simulink model "Host"  (R2024b)
settings: Solver=ode14x  StartTime=0.0  StopTime=inf  FixedStep=hostParams.Ts  RelTol=1e-3
PreLoadFcn:
  | % Load scenario parameters if not already loaded
  | if ~exist('hostParams', 'var')
  |     hostParams = helperScenarioParams;
  | end
  | 
  | % Load vehicle parameters if not already loaded
  | if ~exist('vehicleParams', 'var')
  |     vehicleParams = helperVehicleParams;
  | end
  | 
  | % Load PathFollower parameters if not already loaded
  | if ~exist('controllerParams', 'var')
  |     controllerParams = helperPathFollowerParams;
  | end
  | 
  | % Set IP addresses to local computer if they are not provided
  | if ~exist('ipAddress', 'var')
  |     ipAddress = helperIPAddresses;
  | end
StopFcn:
  | close(gcf)
  | clear functions
libraries: simulink x5, slrealtimeutilitieslib x3, slrealtimeiplib x3, offroadsim3dlib x1, sim3dlib x1, sim3dautolib x1
settings Model: Creator=smaddina  LastModifiedBy=demo-user2
settings SolverCC: PositivePriorityOrder=on
settings OptimizationCC: BlockReduction=off  DefaultParameterBehavior=Inlined  EnhancedBackFolding=on  PassReuseOutputArgsAs=Individual arguments  ZeroExternalMemoryAtStartup=off  ZeroInternalMemoryAtStartup=off  MaxStackSize=64  OptimizeBlockOrder=speed  DifferentSizesBufferReuse=on  OptimizationCustomize=off  EfficientTunableParamExpr=on
settings DebuggingCC: TasksWithSamePriorityMsg=none  ParameterTunabilityLossMsg=error
settings SFSimCC: MATLABDynamicMemAlloc=off
settings RTWCC: Description=Embedded Coder  SystemTargetFile=ert.tlc  TemplateMakefile=ert_default_tmf  Toolchain=Colcon Tools  BuildConfiguration=Faster Runs  CodeExecutionProfiling=on
settings CodeAppCC: ForceParamTrailComments=on  IgnoreCustomStorageClasses=off  MaxIdLength=95  OperatorAnnotations=on  SimulinkDataObjDesc=on  SFDataObjDesc=on  InsertBlockDesc=on
settings ERTTargetCC: RootIOFormat=Structure reference  ERTCustomFileTemplate=example_file_process.tlc

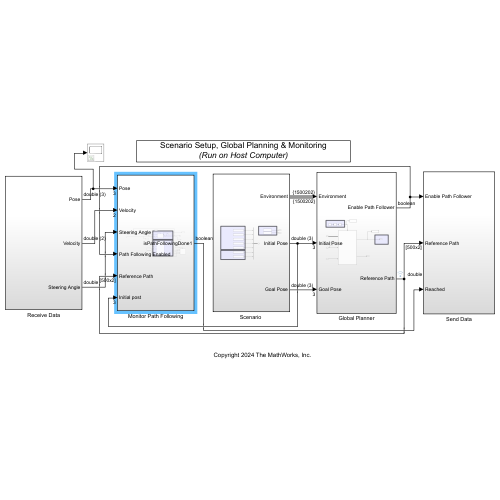
[thumbnail: Simulink's stored preview of the top-level diagram]
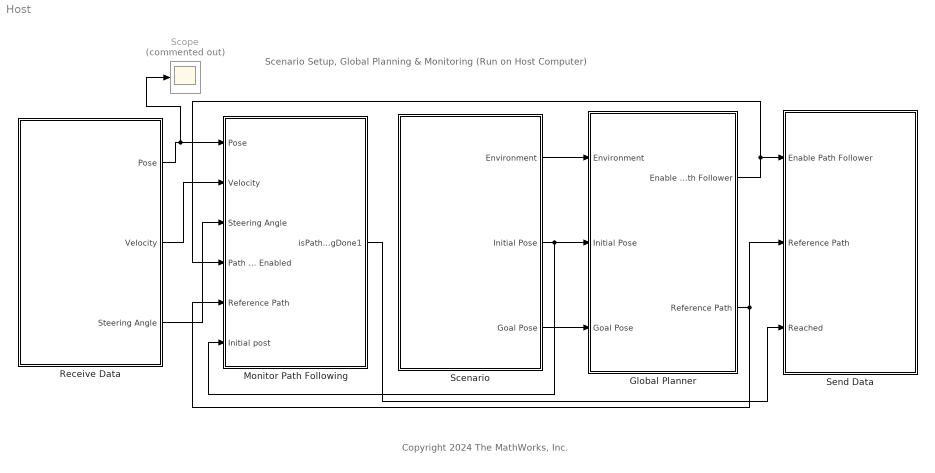
== system Host ==
  note: Copyright 2024 The MathWorks, Inc.
  note: Scenario Setup, Global Planning & Monitoring
      | (Run on Host Computer)
  Global Planner : Subsystem
  Monitor Path Following : Subsystem
  Receive Data : Subsystem
  "Scenario " : Subsystem
  Scope : Scope  Commented=on
  Send Data : Subsystem
  wires:
  Global Planner/2(Reference Path) -> Send Data/2(Reference Path), Monitor Path Following/5(Reference Path)
  Global Planner/1(Enable Path Follower) -> Send Data/1(Enable Path Follower), Monitor Path Following/4(Path Following Enabled)
  "Scenario "/1(Environment) -> Global Planner/1(Environment)
  "Scenario "/2(Initial Pose) -> Monitor Path Following/6(Initial post), Global Planner/2(Initial Pose)
  "Scenario "/3(Goal Pose) -> Global Planner/3(Goal Pose)
  Receive Data/1(Pose) -> Scope/1, Monitor Path Following/1(Pose)
  Receive Data/2(Velocity) -> Monitor Path Following/2(Velocity)
  Receive Data/3(Steering Angle) -> Monitor Path Following/3(Steering Angle)
  Monitor Path Following/1(isPathFollowingDone1) -> Send Data/3(Reached)

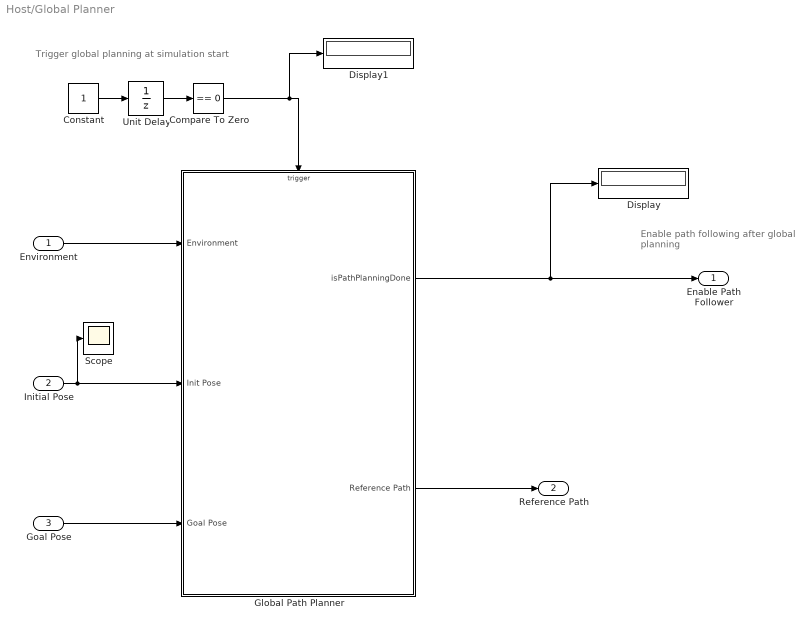
== system Host/Global Planner ==
  note: Enable path following
      | after global planning
  note: Trigger global planning at simulation start
  Environment : Inport
  Initial Pose : Inport  Port=2
  Goal Pose : Inport  Port=3
  Compare To Zero : simulink/Logic and Bit Operations/Compare To Zero  relop===  OutDataTypeStr=boolean
  Constant : Constant
  Display : Display
  Display1 : Display
  Global Path Planner : Subsystem  TreatAsAtomicUnit=on
  Scope : Scope
  Unit Delay : UnitDelay  SampleTime=-1  HasFrameUpgradeWarning=on
  Enable Path Follower : Outport
  Reference Path : Outport  Port=2
  wires:
  Unit Delay/1 -> Compare To Zero/1
  Global Path Planner/2(Reference Path) -> Reference Path/1
  Compare To Zero/1 -> Display1/1, Global Path Planner/Trigger
  Constant/1 -> Unit Delay/1
  Global Path Planner/1(isPathPlanningDone) -> Display/1, Enable Path Follower/1
  Environment/1 -> Global Path Planner/1(Environment)
  Initial Pose/1 -> Scope/1, Global Path Planner/2(Init Pose)
  Goal Pose/1 -> Global Path Planner/3(Goal Pose)

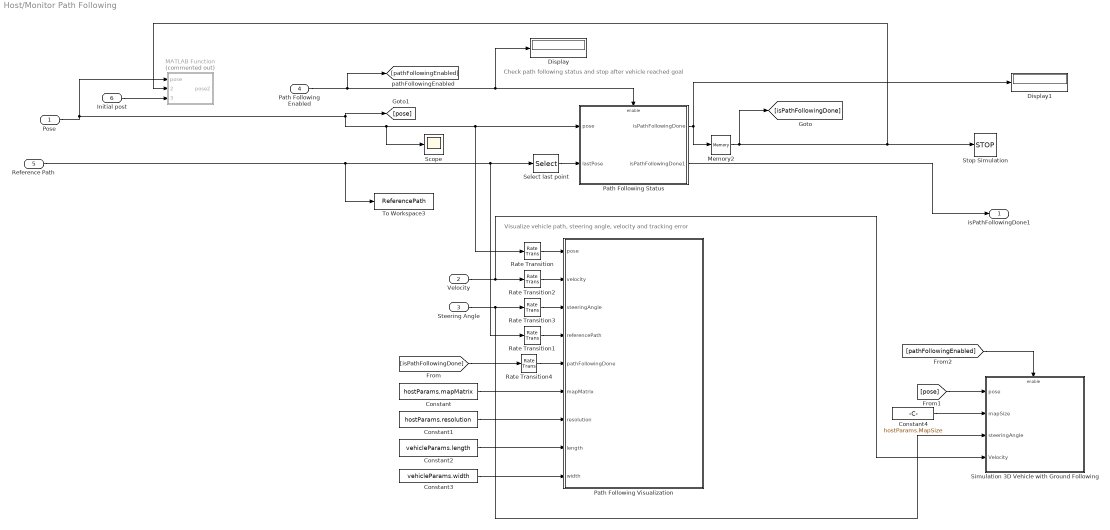
== system Host/Monitor Path Following ==
  note: Visualize vehicle path, steering angle, velocity and tracking error
  note: Check path following status and stop after vehicle reached goal
  Pose : Inport
  Velocity : Inport  Port=2
  Steering Angle : Inport  Port=3
  Path Following Enabled : Inport  Port=4
  Reference Path : Inport  Port=5
  Initial post : Inport  Port=6
  Constant : Constant  Value=hostParams.mapMatrix
  Constant1 : Constant  Value=hostParams.resolution
  Constant2 : Constant  Value=vehicleParams.length
  Constant3 : Constant  Value=vehicleParams.width
  Constant4 : Constant  Value=hostParams.MapSize
  Display : Display
  Display1 : Display
  MATLAB Function : MATLAB Function  Commented=on  TreatAsAtomicUnit=on
  Memory2 : Memory  InitialCondition=false
  Path Following Status : Subsystem
  Path Following Visualization : MATLAB Function  TreatAsAtomicUnit=on  SystemSampleTime=0.2
  Rate Transition : RateTransition  InitialCondition=hostParams.initPose
  Rate Transition1 : RateTransition
  Rate Transition2 : RateTransition
  Rate Transition3 : RateTransition
  Rate Transition4 : RateTransition  InitialCondition=false
  Scope : Scope
  Select last point : Selector  NumberOfDimensions=2  InputPortWidth=3  IndexOptions=Index vector (dialog),Index vector (dialog)  Indices=hostParams.referencePathSize,[1:2]  OutputSizes=1,1
  Simulation 3D Vehicle with Ground Following : Subsystem
  Stop Simulation : Stop
  To Workspace3 : ToWorkspace  VariableName=ReferencePath  SaveFormat=Timeseries  SampleTime=-1
      settings: MaxDataPoints=1
  isPathFollowingDone1 : Outport
  wires:
  Select last point/1 -> Path Following Status/2(lastPose)
  Path Following Status/1(isPathFollowingDone) -> Memory2/1, Display1/1
  Path Following Enabled/1 -> [pathFollowingEnabled], Display/1, Path Following Status/Enable
  Rate Transition/1 -> Path Following Visualization/1(pose)
  Rate Transition1/1 -> Path Following Visualization/4(referencePath)
  Velocity/1 -> Simulation 3D Vehicle with Ground Following/4(Velocity), Rate Transition2/1
  Steering Angle/1 -> Simulation 3D Vehicle with Ground Following/3(steeringAngle), Rate Transition3/1
  Rate Transition2/1 -> Path Following Visualization/2(velocity)
  Rate Transition3/1 -> Path Following Visualization/3(steeringAngle)
  [isPathFollowingDone] -> Rate Transition4/1
  Rate Transition4/1 -> Path Following Visualization/5(pathFollowingDone)
  Constant/1 -> Path Following Visualization/6(mapMatrix)
  Constant1/1 -> Path Following Visualization/7(resolution)
  Constant2/1 -> Path Following Visualization/8(length)
  Constant3/1 -> Path Following Visualization/9(width)
  [pose] -> Simulation 3D Vehicle with Ground Following/1(pose)
  Constant4/1 -> Simulation 3D Vehicle with Ground Following/2(mapSize)
  [pathFollowingEnabled] -> Simulation 3D Vehicle with Ground Following/Enable
  Reference Path/1 -> Select last point/1, Rate Transition1/1, To Workspace3/1
  Pose/1 -> Scope/1, Path Following Status/1(pose), Rate Transition/1, [pose], MATLAB Function/1(pose)
  Initial post/1 -> MATLAB Function/3(initpose)
  Memory2/1 -> Stop Simulation/1, MATLAB Function/2(endoftraj), [isPathFollowingDone]
  Path Following Status/2(isPathFollowingDone1) -> isPathFollowingDone1/1

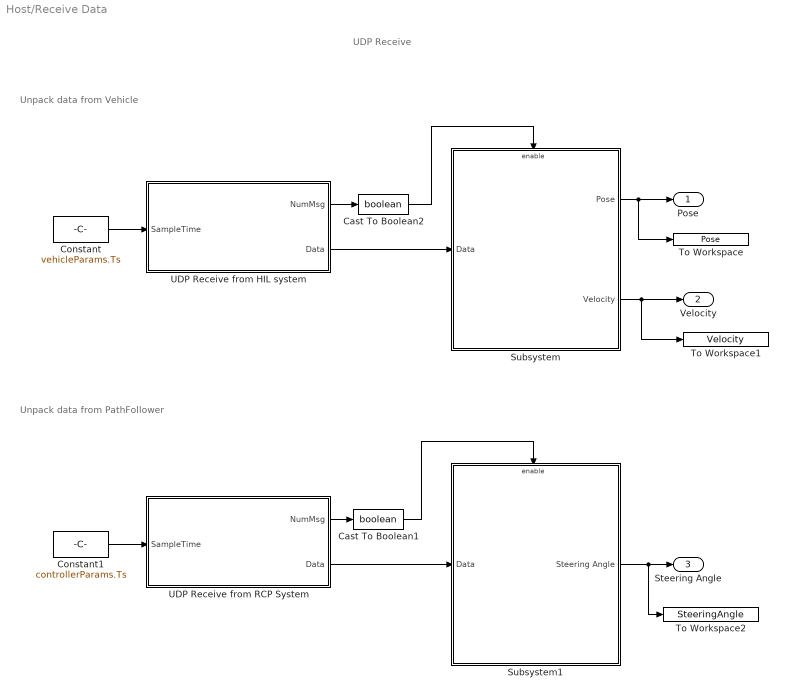
== system Host/Receive Data ==
  note: Unpack data from PathFollower
  note: Unpack data from Vehicle
  note: UDP Receive
  Cast To Boolean1 : DataTypeConversion  OutDataTypeStr=boolean  SaturateOnIntegerOverflow=off  RndMeth=Floor
  Cast To Boolean2 : DataTypeConversion  OutDataTypeStr=boolean  SaturateOnIntegerOverflow=off  RndMeth=Floor
  Constant : Constant  Value=vehicleParams.Ts  SampleTime=vehicleParams.Ts
  Constant1 : Constant  Value=controllerParams.Ts  SampleTime=controllerParams.Ts
  Subsystem : Subsystem
  Subsystem1 : Subsystem
  To Workspace : ToWorkspace  VariableName=Pose  SaveFormat=Timeseries  SampleTime=0.01
  To Workspace1 : ToWorkspace  VariableName=Velocity  SaveFormat=Timeseries  SampleTime=0.01
  To Workspace2 : ToWorkspace  VariableName=SteeringAngle  SaveFormat=Timeseries  SampleTime=0.01
  UDP Receive from HIL system : Subsystem  TreatAsAtomicUnit=on
  UDP Receive from RCP System : Subsystem  TreatAsAtomicUnit=on
  Pose : Outport
  Velocity : Outport  Port=2
  Steering Angle : Outport  Port=3
  wires:
  UDP Receive from HIL system/1(NumMsg) -> Cast To Boolean2/1
  UDP Receive from HIL system/2(Data) -> Subsystem/1(Data)
  Subsystem/1(Pose) -> Pose/1, To Workspace/1
  Subsystem/2(Velocity) -> Velocity/1, To Workspace1/1
  Cast To Boolean2/1 -> Subsystem/Enable
  Subsystem1/1(Steering Angle) -> Steering Angle/1, To Workspace2/1
  Constant/1 -> UDP Receive from HIL system/1(SampleTime)
  UDP Receive from RCP System/2(Data) -> Subsystem1/1(Data)
  Constant1/1 -> UDP Receive from RCP System/1(SampleTime)
  UDP Receive from RCP System/1(NumMsg) -> Cast To Boolean1/1
  Cast To Boolean1/1 -> Subsystem1/Enable

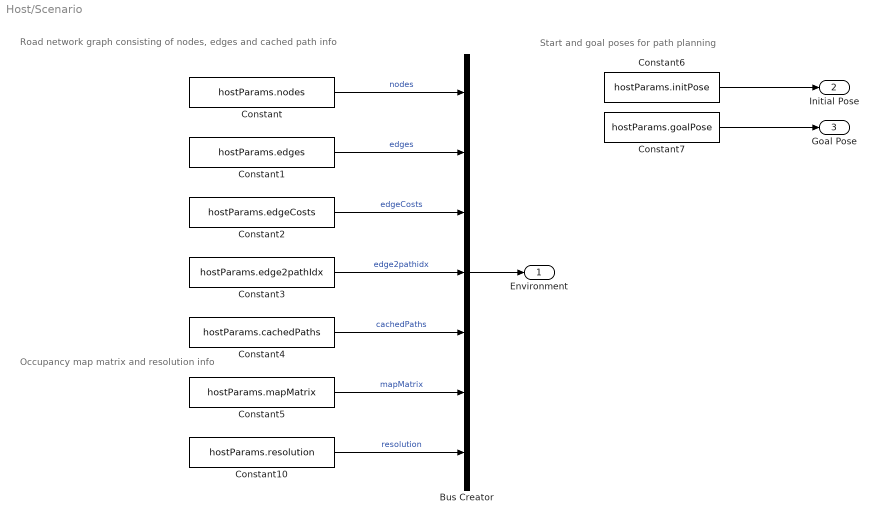
== system Host/Scenario  ==
  note: Start and goal poses for path planning
  note: Occupancy map matrix and
      | resolution info
  note: Road network graph consisting
      | of nodes, edges and cached path info
  Bus Creator : BusCreator  Inputs=7
  Constant : Constant  Value=hostParams.nodes
  Constant1 : Constant  Value=hostParams.edges
  Constant10 : Constant  Value=hostParams.resolution
  Constant2 : Constant  Value=hostParams.edgeCosts
  Constant3 : Constant  Value=hostParams.edge2pathIdx
  Constant4 : Constant  Value=hostParams.cachedPaths
  Constant5 : Constant  Value=hostParams.mapMatrix
  Constant6 : Constant  Value=hostParams.initPose
  Constant7 : Constant  Value=hostParams.goalPose
  Environment : Outport
  Initial Pose : Outport  Port=2
  Goal Pose : Outport  Port=3
  wires:
  Constant/1 -> Bus Creator/1  "nodes"
  Constant1/1 -> Bus Creator/2  "edges"
  Constant2/1 -> Bus Creator/3  "edgeCosts"
  Constant4/1 -> Bus Creator/5  "cachedPaths"
  Constant3/1 -> Bus Creator/4  "edge2pathidx"
  Constant5/1 -> Bus Creator/6  "mapMatrix"
  Constant10/1 -> Bus Creator/7  "resolution"
  Bus Creator/1 -> Environment/1
  Constant7/1 -> Goal Pose/1
  Constant6/1 -> Initial Pose/1

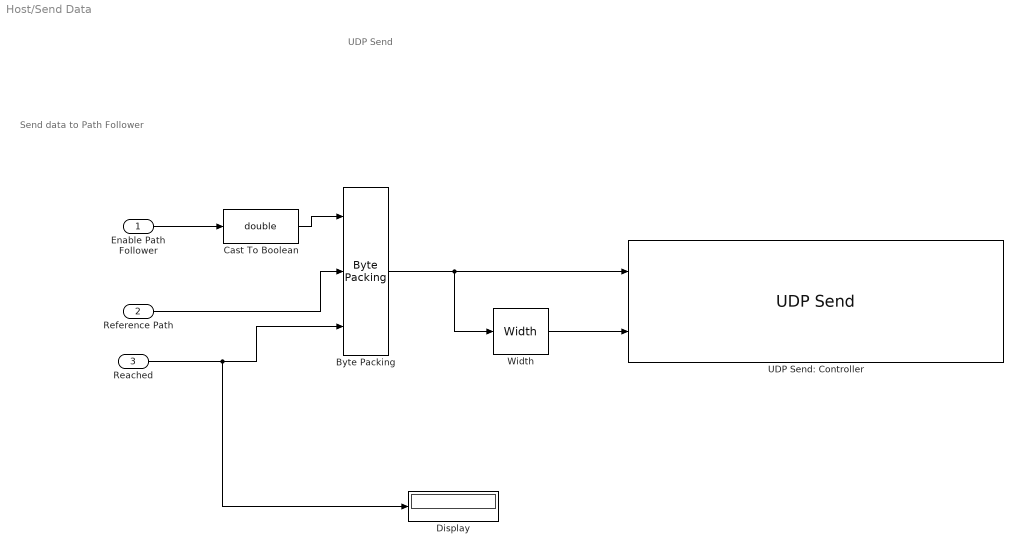
== system Host/Send Data ==
  note: Send data to Path Follower
  note: UDP Send
  Enable Path Follower : Inport
  Reference Path : Inport  Port=2
  Reached : Inport  Port=3
  Byte Packing : slrealtimeutilitieslib/Byte Packing  MaskPackedDataType=uint8  MaskUnpackedDataTypes="{'double',  'double','boolean'}"  MaskAlignment=1
  Cast To Boolean : DataTypeConversion  OutDataTypeStr=double  SaturateOnIntegerOverflow=off  RndMeth=Floor
  Display : Display
  UDP Send: Controller : slrealtimeiplib/UDP Send  useHostTargetConn=on  toAddress=ipAddress.rcpSystem  toPort=8001  sampleTime=-1  enableMessage=off  localPort=-1
  Width : Width
  wires:
  Width/1 -> UDP Send: Controller/2
  Byte Packing/1 -> UDP Send: Controller/1, Width/1
  Reference Path/1 -> Byte Packing/2
  Enable Path Follower/1 -> Cast To Boolean/1
  Cast To Boolean/1 -> Byte Packing/1
  Reached/1 -> Display/1, Byte Packing/3

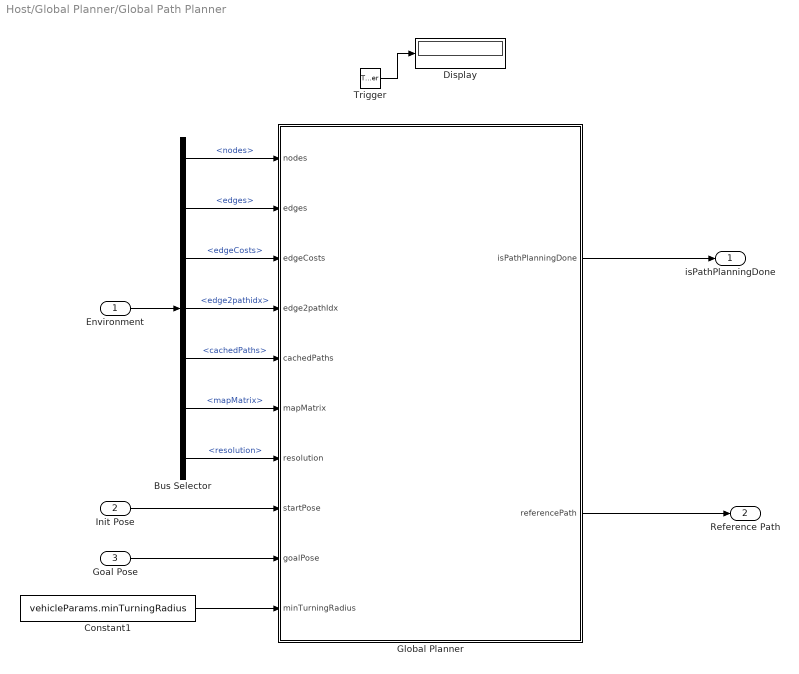
== system Host/Global Planner/Global Path Planner ==
  Environment : Inport
  Init Pose : Inport  Port=2
  Goal Pose : Inport  Port=3
  Trigger : TriggerPort  TriggerType=falling  VariantControl=(inherit)  ShowOutputPort=on  PortDimensions=1
  Bus Selector : BusSelector  OutputSignals=nodes,edges,edgeCosts,edge2pathidx,cachedPaths,mapMatrix,resolution
  Constant1 : Constant  Value=vehicleParams.minTurningRadius
  Display : Display
  Global Planner : MATLAB Function  InitFcn=referencePathSize = hostParams.referencePathSize;  TreatAsAtomicUnit=on
  isPathPlanningDone : Outport
  Reference Path : Outport  Port=2
  wires:
  Global Planner/1(isPathPlanningDone) -> isPathPlanningDone/1
  Global Planner/2(referencePath) -> Reference Path/1
  Environment/1 -> Bus Selector/1
  Bus Selector/2 -> Global Planner/2(edges)  "<edges>"
  Bus Selector/1 -> Global Planner/1(nodes)  "<nodes>"
  Bus Selector/3 -> Global Planner/3(edgeCosts)  "<edgeCosts>"
  Bus Selector/4 -> Global Planner/4(edge2pathIdx)  "<edge2pathidx>"
  Bus Selector/5 -> Global Planner/5(cachedPaths)  "<cachedPaths>"
  Bus Selector/6 -> Global Planner/6(mapMatrix)  "<mapMatrix>"
  Bus Selector/7 -> Global Planner/7(resolution)  "<resolution>"
  Init Pose/1 -> Global Planner/8(startPose)
  Goal Pose/1 -> Global Planner/9(goalPose)
  Constant1/1 -> Global Planner/10(minTurningRadius)
  Trigger/1 -> Display/1

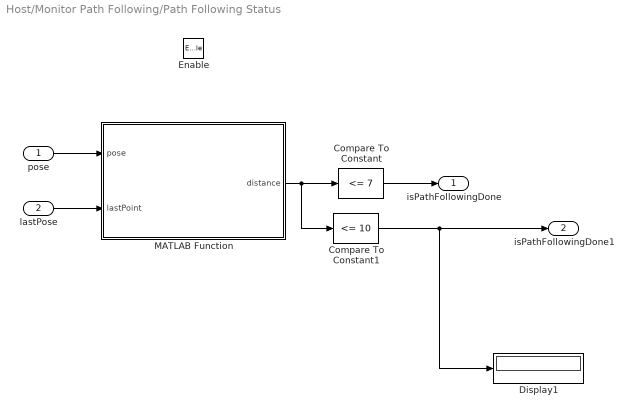
== system Host/Monitor Path Following/Path Following Status ==
  pose : Inport
  lastPose : Inport  Port=2
  Enable : EnablePort
  Compare To Constant : simulink/Logic and Bit Operations/Compare To Constant  relop=<=  const=7  OutDataTypeStr=boolean
  Compare To Constant1 : simulink/Logic and Bit Operations/Compare To Constant  relop=<=  const=10  OutDataTypeStr=boolean
  Display1 : Display
  MATLAB Function : MATLAB Function  TreatAsAtomicUnit=on
  isPathFollowingDone : Outport
  isPathFollowingDone1 : Outport  Port=2
  wires:
  lastPose/1 -> MATLAB Function/2(lastPoint)
  pose/1 -> MATLAB Function/1(pose)
  Compare To Constant/1 -> isPathFollowingDone/1
  MATLAB Function/1(distance) -> Compare To Constant1/1, Compare To Constant/1
  Compare To Constant1/1 -> Display1/1, isPathFollowingDone1/1

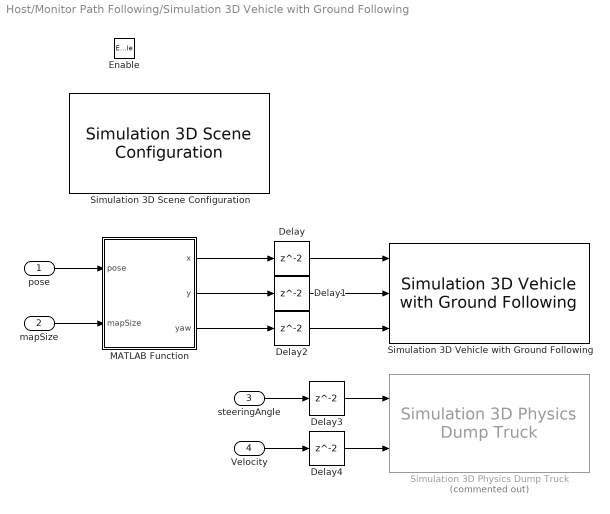
== system Host/Monitor Path Following/Simulation 3D Vehicle with Ground Following ==
  pose : Inport
  mapSize : Inport  Port=2
  steeringAngle : Inport  Port=3
  Velocity : Inport  Port=4
  Enable : EnablePort
  Delay{,1..4} (5 alike) : Delay
  MATLAB Function : MATLAB Function  TreatAsAtomicUnit=on
  Simulation 3D Physics Dump Truck : offroadsim3dlib/Simulation 3D Physics Dump Truck  Commented=on  TruckType=Standard Dump Truck  TruckColor=Yellow  ActorName=SimulinkVehicle2  InitTruckTrans=[0 0 0]  InitTruckRot=[0 0 0]  InitTruckVel=0  InitTruckAccel=0  InitTruckBedAng=0  EnbAccelInp=off  EnbFootBrakInp=off  EnbLifAngInp=off  EnbTruckTransOut=off  EnbTruckRotOut=off  EnbTruckVelOut=off  EnbTruckAngVelOut=off  EnbTruckBedTransOut=off  EnbTruckBedRotOut=off  EnbTruckBedAngOut=off  SampleTime=0.01  ActorType=SimulinkVehicle  ID=2  aMode=6  ActorTag=SimulinkVehicle2  Mesh=DumpTruck
  Simulation 3D Scene Configuration : sim3dlib/Simulation 3D Scene Configuration  Priority=0  ProjectFormat=Default Scenes  SceneDesc=Offroad pit mining scene  ProjectName=C:\Program Files\MATLAB\R2024b\toolbox\shared\sim3d_projects\automotive_project_windows\UE\WindowsNoEditor\VehicleSimulation.exe  ScenePath=/Game/Maps/HwStrght  EnableOpenDRIVE=off  vehTagList={'Custom';'Scene Origin';'SimulinkVehicle1'}  vehTag=SimulinkVehicle1  FreeCameraInitialTranslation=[0, 0, 0]  FreeCameraDefaultInitialTranslation=[-6, 0, 2]  FreeCameraInitialRotation=[0, 0, 0]  FreeCameraDefaultInitialRotation=[0, -15, 0]  OpVisEn=off  Ts=0.02  EnableWindow=on  EnableRemoteAccess=off  EnableWeather=off  SunAzimuth=90  SunAltitude=40.0  EnableGeospatialSun=off  Latitude=0  Longitude=0  Date=2023-01-01  Time=10:30:00  GeoTimeZone=-5.0  SunDaylightSaving=off  wind=1  clouds=10  EnableVolumetricClouds=off  CloudCoverage=0  CloudAltitude=6  fog=0  rain=0  RaindropsEffect=off  SnowDensity=0  EnableGeospatial=off  UseTrueOrigin=off  OriginHeight=200  OriginLatitude=40.744652  OriginLongitude=-73.988864  MapStyle=Aerial  AdditionalAssetIDs=[]  UseAdvancedSunSky=off  SolarTime=11  TimeZone=-5  Day=21  Month=9  Year=2022  UseDaylightSavingTime=on  DSTStartDay=10  DSTStartMonth=3  DSTEndDay=3  DSTEndMonth=11  DSTSwitchHour=2  sensorTag=MainCamera1  sensorId=1  sensorName=MainCamera1  mountLoc=Origin  offsetFlag=off  tmountOffset=[0, 0, 0]  rmountOffset=[0, 0, 0]  HorizontalResolution=1280  VerticalResolution=720  HorizontalFOV=60  mountPoint=[0 0 0]  mountOrientation=[0 0 0]  aMode=6  ID=1  GeoTrigger=Inactive
      settings: LibrarySourceBlock=offroadsim3dlib/Simulation 3D Scene Configuration
  Simulation 3D Vehicle with Ground Following : sim3dautolib/Simulation 3D Vehicle with Ground Following  Priority=1  PassVehMesh=Small pickup truck  MeshPath=/MathWorksAutomotiveContent/Vehicles/Muscle/Meshes/SK_MuscleCar.SK_MuscleCar  TrackWidth=1.9  WheelBase=3  WheelRadius=0.35  VehColor=Red  InitialPos=hostParams.Sim3DInitTranslation  InitialRot=hostParams.Sim3DInitRotation  ActorName=SimulinkVehicle1  SampleTime=hostParams.Ts  ActorType=SimulinkVehicle  ID=1  aMode=5  ActorTag=SimulinkVehicle1  CoordinateScheme=ISO  VehLightsControl=off  HeadlightColor=[ 1, 1, 1 ]  HighBeamIntensity=100000  LowBeamIntensity=60000  HighBeamConeAngle=70  LowBeamConeAngle=70  LeftHeadlightOrientation=[ 0, 0 ]  RightHeadlightOrientation=[ 0, 0 ]  BrakelightIntensity=500  ReverselightIntensity=500  SignallightIntensity=500  SignallightPeriod=1  SignalPulseWidth=50  TransformOutportEnabled=off
      settings: LibrarySourceBlock=sl3dlib/Simulation 3D/Actors/Simulation 3D Vehicle with Ground Following
  wires:
  mapSize/1 -> MATLAB Function/2(mapSize)
  pose/1 -> MATLAB Function/1(pose)
  MATLAB Function/1(x) -> Delay/1
  MATLAB Function/2(y) -> Delay1/1
  MATLAB Function/3(yaw) -> Delay2/1
  Delay/1 -> Simulation 3D Vehicle with Ground Following/1
  Delay1/1 -> Simulation 3D Vehicle with Ground Following/2
  Delay2/1 -> Simulation 3D Vehicle with Ground Following/3
  steeringAngle/1 -> Delay3/1
  Velocity/1 -> Delay4/1
  Delay3/1 -> Simulation 3D Physics Dump Truck/1
  Delay4/1 -> Simulation 3D Physics Dump Truck/2

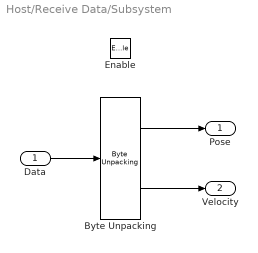
== system Host/Receive Data/Subsystem ==
  Data : Inport
  Enable : EnablePort
  Byte Unpacking : slrealtimeutilitieslib/Byte Unpacking  MaskUnpackedDataTypes={ 'double', 'double'}  MaskUnpackedDataSizes={3, 2}  MaskAlignment=1
  Pose : Outport
  Velocity : Outport  Port=2
  wires:
  Byte Unpacking/2 -> Velocity/1
  Data/1 -> Byte Unpacking/1
  Byte Unpacking/1 -> Pose/1

== system Host/Receive Data/Subsystem1 ==
  Data : Inport
  Enable : EnablePort
  Acceleration : Terminator
  Byte Unpacking : slrealtimeutilitieslib/Byte Unpacking  MaskUnpackedDataTypes="{'double',  'double'}"  MaskUnpackedDataSizes={1, 1}  MaskAlignment=1
  Steering Angle : Outport
  wires:
  Data/1 -> Byte Unpacking/1
  Byte Unpacking/2 -> Steering Angle/1
  Byte Unpacking/1 -> Acceleration/1

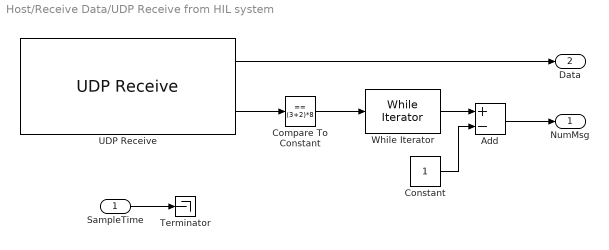
== system Host/Receive Data/UDP Receive from HIL system ==
  SampleTime : Inport
  Add : Sum  Inputs=+-
  Compare To Constant : simulink/Logic and Bit Operations/Compare To Constant  relop===  const=(3+2)*8  OutDataTypeStr=boolean
  Constant : Constant
  Terminator : Terminator
  UDP Receive : slrealtimeiplib/UDP Receive  useHostTargetConn=on  ipAddress=10.10.10.15  localPort=8005  rcvWidth=(3+2)*8  rcvFmAny=on  fmAddress='10.10.10.10'  sampleTime=-1  enableMessage=off  maxPackets=1
  While Iterator : WhileIterator  WhileBlockType=do-while  ShowIterationPort=on
  NumMsg : Outport
  Data : Outport  Port=2
  wires:
  Compare To Constant/1 -> While Iterator/1
  UDP Receive/1 -> Data/1
  UDP Receive/2 -> Compare To Constant/1
  Add/1 -> NumMsg/1
  While Iterator/1 -> Add/1
  Constant/1 -> Add/2
  SampleTime/1 -> Terminator/1

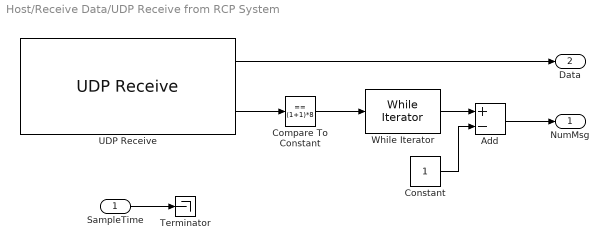
== system Host/Receive Data/UDP Receive from RCP System ==
  SampleTime : Inport
  Add : Sum  Inputs=+-
  Compare To Constant : simulink/Logic and Bit Operations/Compare To Constant  relop===  const=(1+1)*8  OutDataTypeStr=boolean
  Constant : Constant
  Terminator : Terminator
  UDP Receive : slrealtimeiplib/UDP Receive  useHostTargetConn=on  ipAddress=10.10.10.15  localPort=8004  rcvWidth=(1+1)*8  rcvFmAny=on  fmAddress='10.10.10.10'  sampleTime=-1  enableMessage=off  maxPackets=1
  While Iterator : WhileIterator  WhileBlockType=do-while  ShowIterationPort=on
  NumMsg : Outport
  Data : Outport  Port=2
  wires:
  Compare To Constant/1 -> While Iterator/1
  UDP Receive/1 -> Data/1
  UDP Receive/2 -> Compare To Constant/1
  Add/1 -> NumMsg/1
  While Iterator/1 -> Add/1
  Constant/1 -> Add/2
  SampleTime/1 -> Terminator/1

== matlab function Host/Global Planner/Global Path Planner/Global Planner ==
  data: isPathPlanningDone output; nodes input; edges input; edgeCosts input; edge2pathIdx input; cachedPaths input; mapMatrix input; resolution input; startPose input; goalPose input; referencePath output size=[hostParams.referencePathSize,2]; minTurningRadius input; referencePathSize parameter
function [isPathPlanningDone, referencePath] = planRoadNetworkPath(...
    nodes, edges, edgeCosts, edge2pathIdx, cachedPaths,...
    mapMatrix, resolution, startPose, goalPose, minTurningRadius, referencePathSize)

referencePath = zeros(referencePathSize,2);
coder.extrinsic('helperPlanRoadNetworkPath')
out =  helperPlanRoadNetworkPath(nodes, edges, edgeCosts, edge2pathIdx, cachedPaths,...
    mapMatrix, resolution, referencePathSize, minTurningRadius, startPose, goalPose);
referencePath = out;
isPathPlanningDone = true;

== matlab function Host/Monitor Path Following/Path Following Status/MATLAB Function ==
  data: pose input size=[1,3]; distance output; lastPoint input size=[1,2]
function distance = distanceToGoal(pose, lastPoint)

distance = nav.algs.distanceEuclidean(pose([1,2]), lastPoint([1,2]));

== matlab function Host/Monitor Path Following/Simulation 3D Vehicle with Ground Following/MATLAB Function ==
  data: x output; pose input; y output; mapSize input; yaw output
function [x,y,yaw] = fcn(pose, mapSize)

x = pose(1)-mapSize(1)/2;
y = pose(2)-mapSize(2)/2;
yaw = pose(3)*180/pi;

== matlab function Host/Monitor Path Following/Path Following Visualization ==
  data: pose input; velocity input; steeringAngle input; referencePath input; pathFollowingDone input; mapMatrix input; resolution input; length input; width input
function visualizePathFollowing(pose, velocity, steeringAngle, referencePath, pathFollowingDone, mapMatrix, resolution, length, width)
% visualizePathFollowing  Visualize the vehicle trajectory on the occupancy
% map, and other variables such as velocity, steering angle and tracking
% error.
%
%  Note: The vehicle at a given pose will be plotted as a rectangle of
%  dimensions [length, width]

% Copyright 2024 The MathWorks, Inc.

arguments
    % Vehicle pose
    pose (1,3) double

    % Vehicle velocity
    velocity (1,2) double

    % Steering angle
    steeringAngle (1,1) double

    % Reference path to be followed
    referencePath (:,2) double

    % Flag indicating if path following done
    pathFollowingDone (1,1) logical

    % Occupancy grid matrix of the obstacles
    mapMatrix (:,:) logical
    
    % Resolution of the occupancy grid map
    resolution (1,1) double

    % Length of the vehicle
    length (1,1) double
    
    % Width of the vehicle
    width (1,1) double
end

bufferSize = 10000;
coder.extrinsic('plot', 'show', 'fill', 'binaryOccupancyMap')


persistent Step % Step counter
persistent Distance Pose SteeringAngle Velocity TrackingError; % Accumulated data from each time step
persistent axReferencePath axPose axVertices axVelocity axSteeringAngle axTrackingError; % Axes handles
vertices = vehicleVerticies(pose, length, width);

%--------------------------------------------------------------------------
% Create plot for the first time step and store the handles
%--------------------------------------------------------------------------
if isempty(Pose)
    % Create buffer to store simulation data    
    Pose = nan(bufferSize,2);
    Distance = nan(bufferSize, 1);
    Velocity = nan(bufferSize, 1);
    SteeringAngle = nan(bufferSize, 1);
    TrackingError = nan(bufferSize, 1);

    % Update first point data
    Step = 1;
    Pose(1,:) = pose(1:2);
    Distance(1) = 0;
    Velocity(1) = velocity(1);
    SteeringAngle(1) = 0;
    TrackingError(1) = 0;

    % Trajectory plot    
    ax1 = subplot(1, 2, 1);
    map = binaryOccupancyMap(mapMatrix, resolution); % Assume map does not change
    show(map);
    hold on
    axReferencePath = plot(referencePath(:,1), referencePath(:,2), LineWidth=2, Color="#0072BD");
    axPose = plot(pose(1), pose(2), LineWidth=2, Color="#D95319");
    legend([axReferencePath,axPose], {'Reference Path', 'Actual Path'})
    axVertices = fill(vertices(:,1), vertices(:,2), [0.466 0.674 0.188], 'FaceAlpha', 0.7); % Fill with light red    
    set(get(get(axVertices, 'Annotation'), 'LegendInformation'), 'IconDisplayStyle', 'off');

    % Velocity plot
    subplot(3, 2, 2)
    axVelocity = plot(0, velocity(1));
    title('Linear Velocity [m/s]')

    % Steering angle plot
    subplot(3, 2, 4)
    axSteeringAngle = plot(0, steeringAngle);
    title('Steering Angle [rad]')

    % Tracking error plot
    subplot(3, 2, 6)
    axTrackingError = plot(0, 0);
    title('Tracking Error [m]')
    
    axes(ax1) % Make trajectory plot axes as the active one
    return
end

%--------------------------------------------------------------------------
% Update plot during the simulation
%--------------------------------------------------------------------------

% Update plot during the simulation
Step = Step + 1;

% Set reference path only once during the simulation when it becomes
% available after the first step
if Step==2
    set(axReferencePath, XData=referencePath(:,1), YData=referencePath(:,2))
end

% Extend memory if bufferSize is exceeded
% if Step == bufferSize
%     Pose = [Pose; nan(bufferSize,2)];
%     Distance = [Distance; nan(bufferSize,1)];
%     Velocity = [Velocity; nan(bufferSize,1)];
%     SteeringAngle = [SteeringAngle; nan(bufferSize,1)];
%     TrackingError = [TrackingError; nan(bufferSize,1)];
% end

% Update persistent variables with current time step data
Pose(Step,:) = pose(1:2);
Distance(Step) = Distance(Step-1) + hypot(pose(1)-Pose(Step-1,1), pose(2)-Pose(Step-1,2));
Velocity(Step) = velocity(1);
SteeringAngle(Step) = steeringAngle;
TrackingError(Step) = min(hypot(referencePath(:,1)-pose(1), referencePath(:,2)-pose(2)));

% Update trajectory plot
set(axPose, XData=Pose(1:Step,1), YData=Pose(1:Step,2));
set(axVertices, XData=vertices(:,1), YData=vertices(:,2));
if ~pathFollowingDone
    xlim([pose(1)-100, pose(1)+100])
    ylim([pose(2)-100, pose(2)+100])
else
    % Reset axes limits
    axes auto
end

% Update velocity, steering angle and tracking error plots 
set(axVelocity, XData=Distance, yData=Velocity);
set(axSteeringAngle, XData=Distance, yData=SteeringAngle);
set(axTrackingError, XData=Distance, yData=TrackingError);
end

function vertices = vehicleVerticies(pose, length, width)
% Corners of the vehicle rectangle
vertices = 0.5*[-1,-1; -1,1; 1,1; 1,-1; -1,-1].*[length, width];

% Rotation matrix
R = [cos(pose(3)), -sin(pose(3)); sin(pose(3)), cos(pose(3))];

% Rotate the rectangle corners
vertices = (R * vertices')';

% Adjust for the center if it's not at the origin
vertices = vertices + pose(1:2);
end

== matlab function Host/Monitor Path Following/MATLAB Function ==
  data: pose input; pose2 output; endoftraj input; initpose input
function pose2 = fcn(pose,endoftraj, initpose)
%#codegen
if endoftraj
    pose2 = initpose;
else
    pose2 = pose;
end

end
